simulink model "sra1"  (R2016a)
settings: Solver=ode45  StartTime=0.0  StopTime=30  RelTol=1e-5
libraries: simulink x1
settings Model: Creator=andrei  LastModifiedBy=andrei

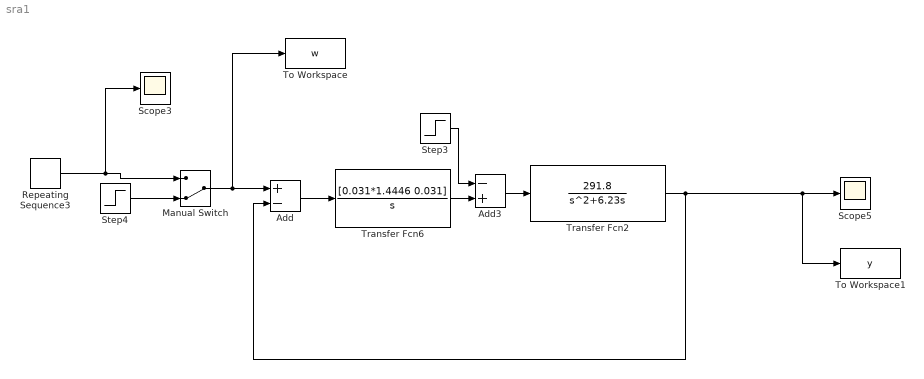
== system sra1 ==
  Add : Sum  Inputs=+-
  Add3 : Sum  Inputs=-+
  Manual Switch : ManualSwitch  CurrentSetting=0
  Repeating Sequence3 : simulink/Sources/Repeating Sequence  rep_seq_t=[0.0001 5 5.0001 10 10.0001]  rep_seq_y=[0.0001 0.0000 5 5 5]
  Scope3 : Scope
  Scope5 : Scope
  Step3 : Step  Time=7.5  After=0.01  SampleTime=0
  Step4 : Step  Time=0  SampleTime=0
  To Workspace : ToWorkspace  VariableName=w  SaveFormat=Timeseries  SampleTime=-1
  To Workspace1 : ToWorkspace  VariableName=y  SaveFormat=Timeseries  SampleTime=-1
  Transfer Fcn2 : TransferFcn  Numerator=[291.8]  Denominator=[1 6.23 0]
  Transfer Fcn6 : TransferFcn  Numerator=[0.031*1.4446 0.031]  Denominator=[1 0]
  wires:
  Add/1 -> Transfer Fcn6/1
  Transfer Fcn2/1 -> Add/2, To Workspace1/1, Scope5/1
  Add3/1 -> Transfer Fcn2/1
  Transfer Fcn6/1 -> Add3/2
  Step3/1 -> Add3/1
  Manual Switch/1 -> To Workspace/1, Add/1
  Step4/1 -> Manual Switch/2
  Repeating Sequence3/1 -> Scope3/1, Manual Switch/1
